simulink library "DodecaPreprocessingLib"  (R2020b)
settings: Solver=VariableStepAuto  StartTime=0.0  StopTime=10.0  RelTol=1e-3
undefined symbols (not defined in the file or in its folder): C_AccFiltCoeff, C_AngleScaleCoeff, C_DirectionTransmissionFactor, C_FiltStWhAngCoeff, C_FiltStWhAngSpdCoeff, C_Te_PPR, C_VehSpdCoeff, C_VspeedWfyaw, C_Wfyaw, C_WheelAxleDistance, N_AccMax, N_AccMin, N_ANGLES_N360_360, N_deg, N_max, N_min, N_pi, N_SIN_REL_N360_360, N_spd_conv
libraries: simulink x8, Valeo_Simulink_Library_EC x4
settings Model: Creator=ahashem  LastModifiedBy=ahashem

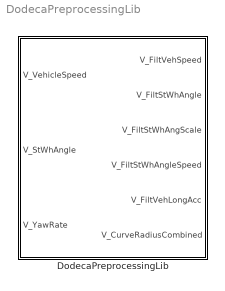
== system DodecaPreprocessingLib ==
  DodecaPreprocessingLib : Subsystem

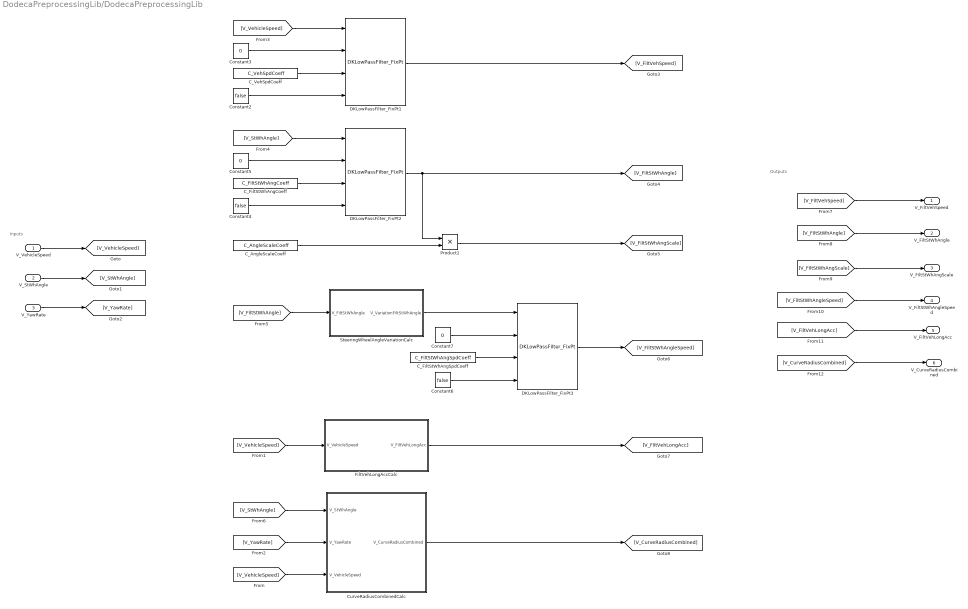
== system DodecaPreprocessingLib/DodecaPreprocessingLib ==
  note: Inputs
  note: Outputs
  V_VehicleSpeed : Inport  RequirementInfo={} %GIDa_60832143_23e3_4e37_9ef8_f4c8fbc195ea
  V_StWhAngle : Inport  RequirementInfo={} %GIDa_8126107c_488a_4046_91e4_66b596814474  Port=2
  V_YawRate : Inport  RequirementInfo={} %GIDa_21efb593_fe6a_4a8c_ad86_ea0a548e14f1  Port=3
  C_AngleScaleCoeff : Constant  RequirementInfo={} %GIDa_0cdad353_1e9f_40d8_8c36_6ad926c040fa  Value=C_AngleScaleCoeff  SampleTime=-1
  C_FiltStWhAngCoeff : Constant  RequirementInfo={} %GIDa_ea71535c_fca6_4d74_a353_bf553c7836cd  Value=C_FiltStWhAngCoeff  SampleTime=-1
  C_FiltStWhAngSpdCoeff : Constant  RequirementInfo={} %GIDa_088bdebb_9f79_46eb_9893_bd4dbe5423a2  Value=C_FiltStWhAngSpdCoeff  SampleTime=-1
  C_VehSpdCoeff : Constant  RequirementInfo={} %GIDa_c5f62ab8_0a9f_4fa0_82aa_9620af8d284b  Value=C_VehSpdCoeff  SampleTime=-1
  Constant2 : Constant  RequirementInfo={} %GIDa_f5b0f010_a49c_40bd_ade5_4da1f284b015  Value=false
  Constant3 : Constant  RequirementInfo={} %GIDa_bbc6fc55_9231_4124_a586_b78e3b3f8e3b  Value=0  OutDataTypeStr=Inherit: Inherit via back propagation
  Constant4 : Constant  RequirementInfo={} %GIDa_8db6b81b_f55b_4d76_a4c4_0f30a2bf3151  Value=false
  Constant5 : Constant  RequirementInfo={} %GIDa_1fff04a1_583c_4fc9_904f_aa895289aece  Value=0  OutDataTypeStr=Inherit: Inherit via back propagation
  Constant6 : Constant  RequirementInfo={} %GIDa_8cf859df_d5fb_4c8d_944a_ef0bb45c25e9  Value=false
  Constant7 : Constant  RequirementInfo={} %GIDa_d8cd6144_71a6_42bf_bf34_bb68e5da6881  Value=0  OutDataTypeStr=Inherit: Inherit via back propagation
  CurveRadiusCombinedCalc : Subsystem  RequirementInfo={} %GIDa_64336f43_2055_4d12_b781_db850783e38b
  DKLowPassFilter_FixPt1 : Valeo_Simulink_Library_EC/Signal_Operations/DKLowPassFilter_FixPt  Description=DKLowPassFilter_FixPt
  DKLowPassFilter_FixPt2 : Valeo_Simulink_Library_EC/Signal_Operations/DKLowPassFilter_FixPt  Description=DKLowPassFilter_FixPt
  DKLowPassFilter_FixPt3 : Valeo_Simulink_Library_EC/Signal_Operations/DKLowPassFilter_FixPt  Description=DKLowPassFilter_FixPt
  FiltVehLongAccCalc : Subsystem  RequirementInfo={} %GIDa_cd813895_0fe0_49b9_8029_c65e3c884f98  TreatAsAtomicUnit=on
  Product1 : Product  RequirementInfo={} %GIDa_f1608e0b_bb6d_46d5_89b0_19cc4592d5c7  OutDataTypeStr=Inherit: Inherit via back propagation  RndMeth=Round
  SteeringWheelAngleVariationCalc : Subsystem  RequirementInfo={} %GIDa_4c57f141_03ad_4307_827e_b71fe2f80d30
  V_FiltVehSpeed : Outport  RequirementInfo={} %GIDa_d767c948_d5f1_431d_a4d9_613e959d2370  VectorParamsAs1DForOutWhenUnconnected=off
  V_FiltStWhAngle : Outport  RequirementInfo={} %GIDa_20373fde_4aa9_40e5_8d80_7fd2414d965e  Port=2  VectorParamsAs1DForOutWhenUnconnected=off
  V_FiltStWhAngScale : Outport  RequirementInfo={} %GIDa_acd3b80a_9b27_4971_9a5d_d5919bd05f96  Port=3  VectorParamsAs1DForOutWhenUnconnected=off
  V_FiltStWhAngleSpeed : Outport  RequirementInfo={} %GIDa_08f10f9a_4278_41b2_90be_4b2c7de53d89  Port=4  VectorParamsAs1DForOutWhenUnconnected=off
  V_FiltVehLongAcc : Outport  RequirementInfo={} %GIDa_a987007b_cd5d_4cab_a6be_c6cc0e461b96  Port=5  VectorParamsAs1DForOutWhenUnconnected=off
  V_CurveRadiusCombined : Outport  RequirementInfo={} %GIDa_3bd352f3_c991_4ae8_b955_130684fa25fc  Port=6  VectorParamsAs1DForOutWhenUnconnected=off
  wires:
  V_VehicleSpeed/1 -> [V_VehicleSpeed]
  DKLowPassFilter_FixPt2/1 -> [V_FiltStWhAngle], Product1/1
  DKLowPassFilter_FixPt3/1 -> [V_FiltStWhAngleSpeed]
  V_YawRate/1 -> [V_YawRate]
  C_FiltStWhAngCoeff/1 -> DKLowPassFilter_FixPt2/3
  Constant7/1 -> DKLowPassFilter_FixPt3/2
  CurveRadiusCombinedCalc/1(V_CurveRadiusCombined) -> [V_CurveRadiusCombined]
  SteeringWheelAngleVariationCalc/1(V_VariationFiltStWhAngle) -> DKLowPassFilter_FixPt3/1
  Constant3/1 -> DKLowPassFilter_FixPt1/2
  [V_FiltStWhAngScale] -> V_FiltStWhAngScale/1
  [V_VehicleSpeed] -> FiltVehLongAccCalc/1(V_VehicleSpeed)
  [V_CurveRadiusCombined] -> V_CurveRadiusCombined/1
  [V_FiltVehLongAcc] -> V_FiltVehLongAcc/1
  [V_FiltStWhAngle] -> V_FiltStWhAngle/1
  [V_VehicleSpeed] -> CurveRadiusCombinedCalc/3(V_VehicleSpeed)
  Constant5/1 -> DKLowPassFilter_FixPt2/2
  [V_FiltVehSpeed] -> V_FiltVehSpeed/1
  [V_StWhAngle] -> CurveRadiusCombinedCalc/1(V_StWhAngle)
  FiltVehLongAccCalc/1(V_FiltVehLongAcc) -> [V_FiltVehLongAcc]
  [V_YawRate] -> CurveRadiusCombinedCalc/2(V_YawRate)
  Product1/1 -> [V_FiltStWhAngScale]
  V_StWhAngle/1 -> [V_StWhAngle]
  [V_FiltStWhAngle] -> SteeringWheelAngleVariationCalc/1(V_FiltStWhAngle)
  Constant4/1 -> DKLowPassFilter_FixPt2/4
  DKLowPassFilter_FixPt1/1 -> [V_FiltVehSpeed]
  Constant6/1 -> DKLowPassFilter_FixPt3/4
  [V_VehicleSpeed] -> DKLowPassFilter_FixPt1/1
  C_VehSpdCoeff/1 -> DKLowPassFilter_FixPt1/3
  [V_StWhAngle] -> DKLowPassFilter_FixPt2/1
  C_AngleScaleCoeff/1 -> Product1/2
  C_FiltStWhAngSpdCoeff/1 -> DKLowPassFilter_FixPt3/3
  Constant2/1 -> DKLowPassFilter_FixPt1/4
  [V_FiltStWhAngleSpeed] -> V_FiltStWhAngleSpeed/1

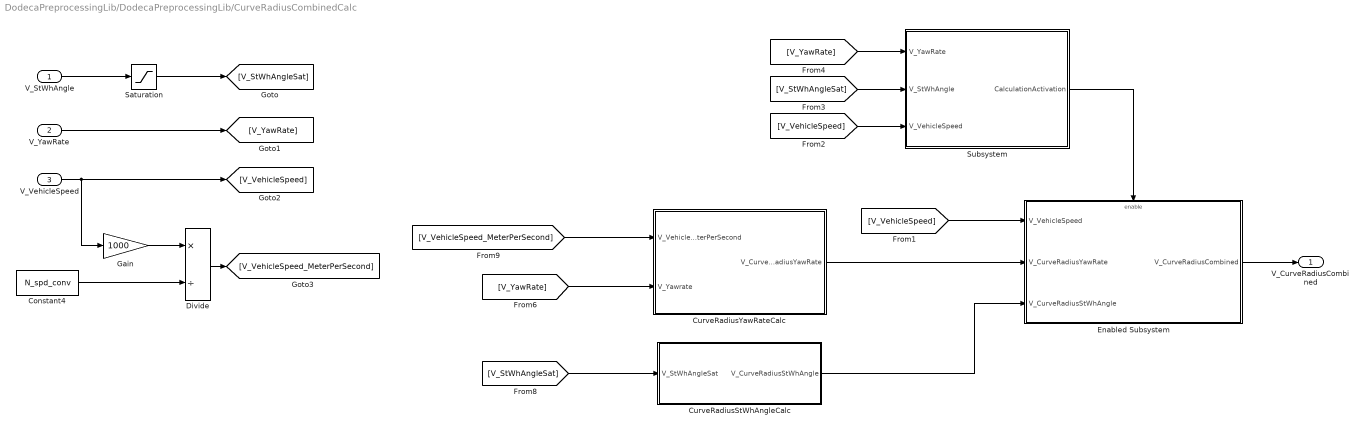
== system DodecaPreprocessingLib/DodecaPreprocessingLib/CurveRadiusCombinedCalc ==
  V_StWhAngle : Inport  RequirementInfo={} %GIDa_c6b31a6f_b3f8_4c38_b982_22111ad8ed9d
  V_YawRate : Inport  RequirementInfo={} %GIDa_7c4cc764_ca2d_41e9_9980_9d9fc3c311cd  Port=2
  V_VehicleSpeed : Inport  RequirementInfo={} %GIDa_23d1c370_e59f_4e6c_b1e1_69d048a5d2a4  Port=3
  Constant4 : Constant  RequirementInfo={} %GIDa_6504d488_faa2_46f4_83bf_1716aa9cad3c  Value=N_spd_conv
  CurveRadiusStWhAngleCalc : Subsystem  RequirementInfo={} %GIDa_d2b816be_039a_44fb_9baa_a094c55a53fb  TreatAsAtomicUnit=on
  CurveRadiusYawRateCalc : Subsystem  RequirementInfo={} %GIDa_2f2fda27_1e9c_44fd_a28d_c3986d892172  TreatAsAtomicUnit=on
  Divide : Product  RequirementInfo={} %GIDa_ae004ed8_02ea_45fd_a30c_5b5e6bbd11bf  Inputs=*/  RndMeth=Nearest
  Enabled Subsystem : Subsystem  RequirementInfo={} %GIDa_f954c3a3_b9a3_4728_bc26_2e3b533776b8  TreatAsAtomicUnit=on
  Gain : Gain  RequirementInfo={} %GIDa_717527a8_c330_4d57_a389_1cff86706634  Gain=1000  OutDataTypeStr=fixdt(1,32,0.01,0)
  Saturation : Saturate  RequirementInfo={} %GIDa_1b87c519_532e_4059_a469_dc5fcda7529d  UpperLimit=360  LowerLimit=-360  OutDataTypeStr=Inherit: Inherit via back propagation
  Subsystem : Subsystem  RequirementInfo={} %GIDa_2fc3370a_ff20_4ea0_b489_573f276c5142
  V_CurveRadiusCombined : Outport  RequirementInfo={} %GIDa_dbce3892_7d57_44c4_a2e6_0566f47b7bcf  VectorParamsAs1DForOutWhenUnconnected=off
  wires:
  Divide/1 -> [V_VehicleSpeed_MeterPerSecond]
  Constant4/1 -> Divide/2
  Gain/1 -> Divide/1
  V_VehicleSpeed/1 -> Gain/1, [V_VehicleSpeed]
  [V_StWhAngleSat] -> CurveRadiusStWhAngleCalc/1(V_StWhAngleSat)
  [V_YawRate] -> CurveRadiusYawRateCalc/2(V_Yawrate)
  [V_VehicleSpeed] -> Enabled Subsystem/1(V_VehicleSpeed)
  Subsystem/1(CalculationActivation) -> Enabled Subsystem/Enable
  [V_YawRate] -> Subsystem/1(V_YawRate)
  [V_StWhAngleSat] -> Subsystem/2(V_StWhAngle)
  [V_VehicleSpeed_MeterPerSecond] -> CurveRadiusYawRateCalc/1("V_VehicleSpeed_MeterPerSecond ")
  V_YawRate/1 -> [V_YawRate]
  Saturation/1 -> [V_StWhAngleSat]
  V_StWhAngle/1 -> Saturation/1
  CurveRadiusYawRateCalc/1(V_CurveRadiusYawRate) -> Enabled Subsystem/2(V_CurveRadiusYawRate)
  CurveRadiusStWhAngleCalc/1(V_CurveRadiusStWhAngle) -> Enabled Subsystem/3(V_CurveRadiusStWhAngle)
  Enabled Subsystem/1(V_CurveRadiusCombined) -> V_CurveRadiusCombined/1
  [V_VehicleSpeed] -> Subsystem/3(V_VehicleSpeed)

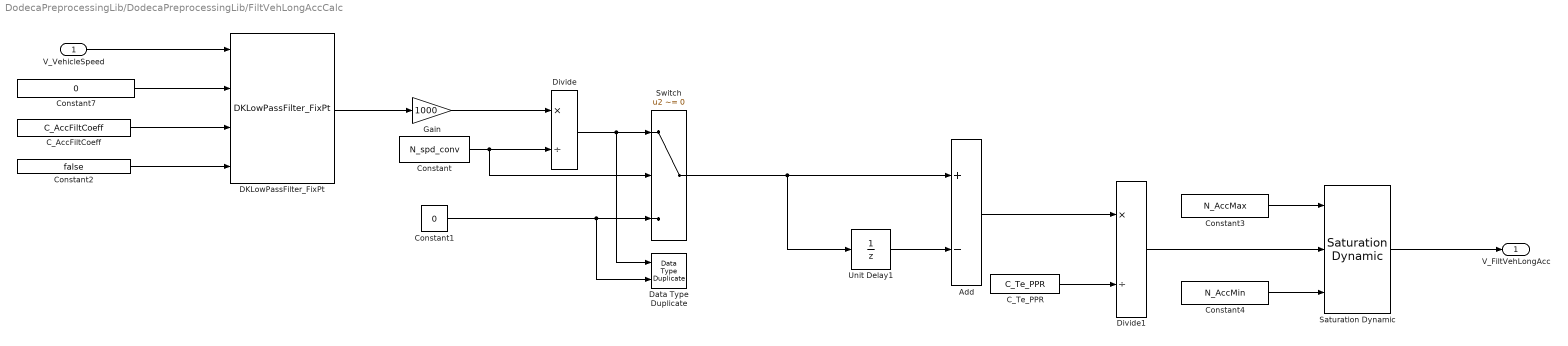
== system DodecaPreprocessingLib/DodecaPreprocessingLib/FiltVehLongAccCalc ==
  V_VehicleSpeed : Inport  RequirementInfo={} %GIDa_a9dff689_ed0f_4809_9958_382473ea2e53
  Add : Sum  RequirementInfo={} %GIDa_b5a1d6ae_d064_4547_8171_96b8d3b4d0ea  Inputs=+-  OutDataTypeStr=Inherit: Inherit via back propagation  RndMeth=Nearest
  C_AccFiltCoeff : Constant  RequirementInfo={} %GIDa_aac16ced_3053_42d0_a1c2_5613f13cadef  Value=C_AccFiltCoeff  SampleTime=-1
  C_Te_PPR : Constant  RequirementInfo={} %GIDa_ca0d0a07_9a87_4e79_85b6_5f4351a4e60f  Value=C_Te_PPR  SampleTime=-1
  Constant : Constant  RequirementInfo={} %GIDa_6440f10a_dfb1_4682_a064_f695864c14d3  Value=N_spd_conv
  Constant1 : Constant  RequirementInfo={} %GIDa_5e43bc7f_985f_4463_932e_96d3615ef032  Value=0  OutDataTypeStr=Inherit: Inherit via back propagation
  Constant2 : Constant  RequirementInfo={} %GIDa_ceee4a21_d10e_4212_9748_3affda2d37ce  Value=false
  Constant3 : Constant  RequirementInfo={} %GIDa_478474b1_827f_4edf_8a52_e111fe7d90da  Value=N_AccMax  VectorParams1D=off  SampleTime=-1
  Constant4 : Constant  RequirementInfo={} %GIDa_dd0b0e05_bb3a_4de4_bc6c_4a6892c59492  Value=N_AccMin  VectorParams1D=off  SampleTime=-1
  Constant7 : Constant  RequirementInfo={} %GIDa_4b056551_402d_41b4_8b01_4fbc664e95cb  Value=0  OutDataTypeStr=Inherit: Inherit via back propagation
  DKLowPassFilter_FixPt : Valeo_Simulink_Library_EC/Signal_Operations/DKLowPassFilter_FixPt  Description=DKLowPassFilter_FixPt
  Data Type Duplicate : DataTypeDuplicate  RequirementInfo={} %GIDa_d4dc3eef_3111_47ac_82d8_48f37c08ca8d
  Divide : Product  RequirementInfo={} %GIDa_2ebbd2e0_80ab_43ba_b182_82a6293abca0  Inputs=*/  RndMeth=Nearest  SaturateOnIntegerOverflow=on  OutDataTypeStr=Inherit: Same as first input
  Divide1 : Product  RequirementInfo={} %GIDa_2bef6155_8d7e_450c_988c_96a89a6309f6  Inputs=*/  OutDataTypeStr=Inherit: Inherit via back propagation  RndMeth=Nearest  SaturateOnIntegerOverflow=on
  Gain : Gain  RequirementInfo={} %GIDa_7eabfaa6_b6cc_4664_8175_45a7b4cb78a3  Gain=1000  OutDataTypeStr=fixdt(1,32,0.0005,0)  RndMeth=Nearest
  Saturation Dynamic : simulink/Discontinuities/Saturation Dynamic  OutMin=[]  OutMax=[]  OutDataTypeStr=fixdt(1,16,0.01,0)  OutputDataTypeScalingMode=Specify via dialog  OutDataType=fixdt(1,16,0.01,0)  OutScaling=[]  DoSatur=off
  Switch : Switch  RequirementInfo={} %GIDa_31131a59_f127_4858_9f67_3213aa90b36b  Criteria=u2 ~= 0
  Unit Delay1 : UnitDelay  RequirementInfo={} %GIDa_5fb9f8c5_fd76_4e8c_b532_a08efb54d5b6  SampleTime=-1  HasFrameUpgradeWarning=on
  V_FiltVehLongAcc : Outport  RequirementInfo={} %GIDa_1047f2a8_4318_4f33_b1e6_f10595ac80de  VectorParamsAs1DForOutWhenUnconnected=off
  wires:
  Constant1/1 -> Switch/3, Data Type Duplicate/2
  Divide/1 -> Switch/1, Data Type Duplicate/1
  Constant/1 -> Divide/2, Switch/2
  C_Te_PPR/1 -> Divide1/2
  Switch/1 -> Unit Delay1/1, Add/1
  Constant3/1 -> Saturation Dynamic/1
  Constant4/1 -> Saturation Dynamic/3
  Gain/1 -> Divide/1
  Add/1 -> Divide1/1
  Constant2/1 -> DKLowPassFilter_FixPt/4
  V_VehicleSpeed/1 -> DKLowPassFilter_FixPt/1
  C_AccFiltCoeff/1 -> DKLowPassFilter_FixPt/3
  Constant7/1 -> DKLowPassFilter_FixPt/2
  DKLowPassFilter_FixPt/1 -> Gain/1
  Unit Delay1/1 -> Add/2
  Divide1/1 -> Saturation Dynamic/2
  Saturation Dynamic/1 -> V_FiltVehLongAcc/1

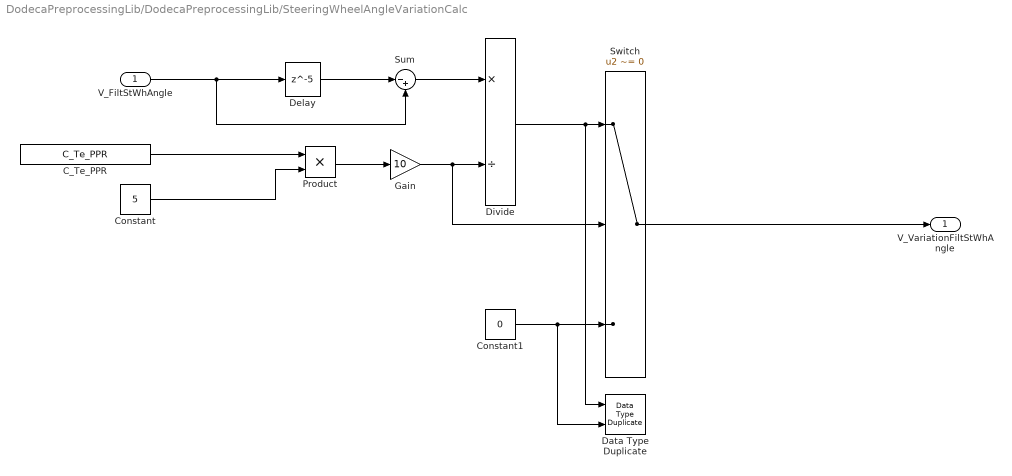
== system DodecaPreprocessingLib/DodecaPreprocessingLib/SteeringWheelAngleVariationCalc ==
  V_FiltStWhAngle : Inport  RequirementInfo={} %GIDa_2d6e10c8_a599_4818_8bca_4fdf95fdb51b
  C_Te_PPR : Constant  RequirementInfo={} %GIDa_d7d2a533_c78c_4824_bc3d_21d571249ced  Value=C_Te_PPR  SampleTime=-1
  Constant : Constant  RequirementInfo={} %GIDa_c4952c67_84f6_4782_887e_253009598a18  Value=5  OutDataTypeStr=uint8
  Constant1 : Constant  RequirementInfo={} %GIDa_c8535ef2_48fc_41db_9114_3d1e05bc0590  Value=0  OutDataTypeStr=Inherit: Inherit via back propagation
  Data Type Duplicate : DataTypeDuplicate  RequirementInfo={} %GIDa_92bb835e_761a_4655_8305_5c552c08e307
  Delay : Delay  RequirementInfo={} %GIDa_72bb8d93_5d0e_4efa_b41a_7b2f3ca524a6  DelayLength=5
  Divide : Product  RequirementInfo={} %GIDa_e876373c_7d20_4d9f_848c_1236b8df3224  Inputs=*/  OutDataTypeStr=Inherit: Inherit via back propagation  RndMeth=Nearest  SaturateOnIntegerOverflow=on
  Gain : Gain  RequirementInfo={} %GIDa_7bda443d_549c_42d1_a512_94fec012033d  Gain=10  OutDataTypeStr=Inherit: Same as input
  Product : Product  RequirementInfo={} %GIDa_d173abd4_ab08_494f_97f9_3c8702ce310b  OutDataTypeStr=Inherit: Same as first input
  Sum : Sum  RequirementInfo={} %GIDa_9d1cd385_e87c_41c8_a3c2_c3015445a319  Inputs=|-+  InputSameDT=on  SaturateOnIntegerOverflow=on  OutDataTypeStr=Inherit: Same as first input
  Switch : Switch  RequirementInfo={} %GIDa_fbe2b111_2dff_405a_b4e7_13e74d307d11  Criteria=u2 ~= 0
  V_VariationFiltStWhAngle : Outport  RequirementInfo={} %GIDa_7cff779a_541a_4368_a5cc_b4cb3fe5e430  VectorParamsAs1DForOutWhenUnconnected=off
  wires:
  Gain/1 -> Divide/2, Switch/2
  Product/1 -> Gain/1
  Switch/1 -> V_VariationFiltStWhAngle/1
  Divide/1 -> Switch/1, Data Type Duplicate/1
  Constant1/1 -> Switch/3, Data Type Duplicate/2
  C_Te_PPR/1 -> Product/1
  Constant/1 -> Product/2
  V_FiltStWhAngle/1 -> Sum/2, Delay/1
  Sum/1 -> Divide/1
  Delay/1 -> Sum/1

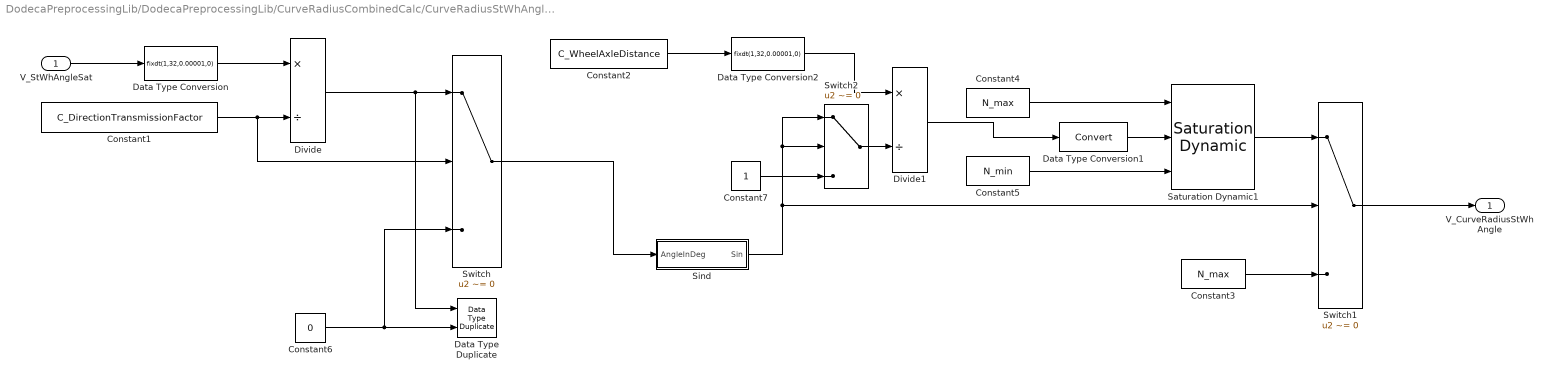
== system DodecaPreprocessingLib/DodecaPreprocessingLib/CurveRadiusCombinedCalc/CurveRadiusStWhAngleCalc ==
  V_StWhAngleSat : Inport  RequirementInfo={} %GIDa_abb681a8_9c5f_45e7_85c6_1a1dee86fac2
  Constant1 : Constant  RequirementInfo={} %GIDa_98570868_5dac_488f_8353_c0564531cf00  Value=C_DirectionTransmissionFactor
  Constant2 : Constant  RequirementInfo={} %GIDa_62b48d84_6a64_4fdc_8bb8_1a0424173a6d  Value=C_WheelAxleDistance
  Constant3 : Constant  Value=N_max
  Constant4 : Constant  RequirementInfo={} %GIDa_fa7813f2_9f7f_4d54_bbcf_f72d7c254580  Value=N_max
  Constant5 : Constant  RequirementInfo={} %GIDa_dd5c7f71_2632_4dc2_942f_60a3de9821df  Value=N_min
  Constant6 : Constant  RequirementInfo={} %GIDa_a1627ed7_883d_4f6e_b8c6_462b0de5ac4d  Value=0  OutDataTypeStr=Inherit: Inherit via back propagation
  Constant7 : Constant  OutDataTypeStr=Inherit: Inherit via back propagation
  Data Type Duplicate : DataTypeDuplicate  RequirementInfo={} %GIDa_9fb6f9e2_a828_4c5c_bf89_f0860357c30f
  Data Type Conversion : DataTypeConversion  RequirementInfo={} %GIDa_2b46cdeb_753e_4edf_9749_a9910cb6b44c  OutDataTypeStr=fixdt(1,32,0.00001,0)
  Data Type Conversion1 : DataTypeConversion  RequirementInfo={} %GIDa_3c386ddb_68dc_423b_897b_b241bf86d79b  RndMeth=Nearest
  Data Type Conversion2 : DataTypeConversion  RequirementInfo={} %GIDa_3ec3c6aa_b003_4747_bc1a_e15dfe0f1686  OutDataTypeStr=fixdt(1,32,0.00001,0)
  Divide : Product  RequirementInfo={} %GIDa_6c6f0a1c_13d3_4619_9e0e_e7ddaa12e435  Inputs=*/  RndMeth=Nearest  SaturateOnIntegerOverflow=on  OutDataTypeStr=Inherit: Same as first input
  Divide1 : Product  RequirementInfo={} %GIDa_1850e6e0_24fb_4802_a9cd_363db8f8d411  Inputs=*/  RndMeth=Nearest  SaturateOnIntegerOverflow=on  OutDataTypeStr=Inherit: Same as first input
  Saturation Dynamic1 : simulink/Discontinuities/Saturation Dynamic  OutMin=[]  OutMax=[]  OutDataTypeStr=int16  OutputDataTypeScalingMode=int16  OutDataType=fixdt(1, 16)  OutScaling=2^-10  DoSatur=off
  Sind : Subsystem  RequirementInfo={} %GIDa_c2fe74d6_4e4e_4053_a67d_4d963e843008
  Switch : Switch  RequirementInfo={} %GIDa_946765d4_88f0_459a_88a2_95c5b5a25c8b  Criteria=u2 ~= 0
  Switch1 : Switch  RequirementInfo={} %GIDa_9d5e6c70_41f5_4b04_9d9f_b48aab403a01  Criteria=u2 ~= 0
  Switch2 : Switch  Criteria=u2 ~= 0
  V_CurveRadiusStWhAngle : Outport  RequirementInfo={} %GIDa_d4150f61_a977_42d0_8013_f59b9b8bd2a2  VectorParamsAs1DForOutWhenUnconnected=off
  wires:
  Data Type Conversion1/1 -> Saturation Dynamic1/2
  Switch1/1 -> V_CurveRadiusStWhAngle/1
  Saturation Dynamic1/1 -> Switch1/1
  Divide1/1 -> Data Type Conversion1/1
  Data Type Conversion2/1 -> Divide1/1
  Constant1/1 -> Divide/2, Switch/2
  Data Type Conversion/1 -> Divide/1
  Divide/1 -> Data Type Duplicate/1, Switch/1
  Constant6/1 -> Switch/3, Data Type Duplicate/2
  Constant5/1 -> Saturation Dynamic1/3
  Constant4/1 -> Saturation Dynamic1/1
  Switch/1 -> Sind/1(AngleInDeg)
  V_StWhAngleSat/1 -> Data Type Conversion/1
  Constant2/1 -> Data Type Conversion2/1
  Sind/1(Sin) -> Switch2/1, Switch2/2, Switch1/2
  Constant3/1 -> Switch1/3
  Switch2/1 -> Divide1/2
  Constant7/1 -> Switch2/3

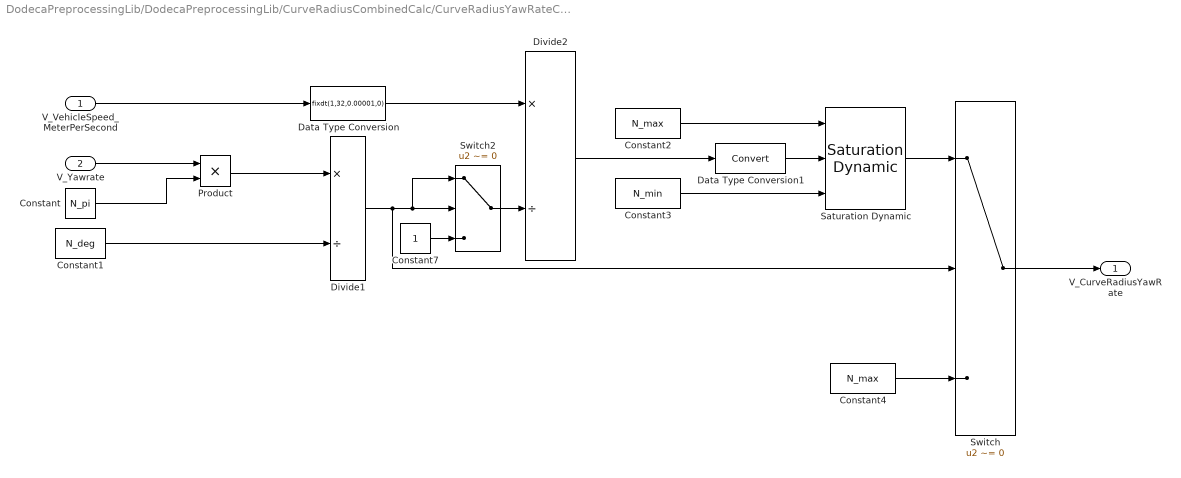
== system DodecaPreprocessingLib/DodecaPreprocessingLib/CurveRadiusCombinedCalc/CurveRadiusYawRateCalc ==
  "V_VehicleSpeed_MeterPerSecond " : Inport  RequirementInfo={} %GIDa_b8150515_5fed_43e7_a020_4c3dd0662e2c
  V_Yawrate : Inport  RequirementInfo={} %GIDa_a8c62ac7_f65c_41a8_8300_229a5a8f87bd  Port=2
  Constant : Constant  RequirementInfo={} %GIDa_5cc06acd_85f2_41c2_868f_dd9dcb282a6d  Value=N_pi
  Constant1 : Constant  RequirementInfo={} %GIDa_0439bdf0_1d9d_4128_851a_8e4062f2ea6e  Value=N_deg
  Constant2 : Constant  RequirementInfo={} %GIDa_9d31224f_c4e5_4964_84c0_bdb99a5399a4  Value=N_max
  Constant3 : Constant  RequirementInfo={} %GIDa_b839a59b_1189_4377_b595_5dfb5ba75ca6  Value=N_min
  Constant4 : Constant  Value=N_max
  Constant7 : Constant  OutDataTypeStr=Inherit: Inherit via back propagation
  Data Type Conversion : DataTypeConversion  RequirementInfo={} %GIDa_bb5325b8_eece_4956_a4e1_c3c780cceb19  OutDataTypeStr=fixdt(1,32,0.00001,0)  RndMeth=Nearest
  Data Type Conversion1 : DataTypeConversion  RequirementInfo={} %GIDa_b72d1d93_d1e7_44eb_9859_a7d629f5b22f  RndMeth=Nearest
  Divide1 : Product  RequirementInfo={} %GIDa_c4f2fba1_a6dc_479b_859e_320a67e827c4  Inputs=*/  RndMeth=Nearest  OutDataTypeStr=Inherit: Same as first input
  Divide2 : Product  RequirementInfo={} %GIDa_3edd98d5_7516_4631_93a5_dc5abed02e4a  Inputs=*/  RndMeth=Nearest  SaturateOnIntegerOverflow=on  OutDataTypeStr=Inherit: Same as first input
  Product : Product  RequirementInfo={} %GIDa_deeedb41_50b5_400e_a3b1_edb035b115c2  OutDataTypeStr=fixdt(1,32,0.00001,0)  RndMeth=Nearest
  Saturation Dynamic : simulink/Discontinuities/Saturation Dynamic  OutMin=[]  OutMax=[]  OutDataTypeStr=int16  OutputDataTypeScalingMode=int16  OutDataType=fixdt(1, 16)  OutScaling=2^-10  DoSatur=off
  Switch : Switch  RequirementInfo={} %GIDa_9386fa3b_9e9d_48a1_80ed_e0e569d2533b  Criteria=u2 ~= 0
  Switch2 : Switch  Criteria=u2 ~= 0
  V_CurveRadiusYawRate : Outport  RequirementInfo={} %GIDa_8a4eb58c_61b4_43a7_81c7_927a1839a6fd  VectorParamsAs1DForOutWhenUnconnected=off
  wires:
  Data Type Conversion1/1 -> Saturation Dynamic/2
  Saturation Dynamic/1 -> Switch/1
  Switch/1 -> V_CurveRadiusYawRate/1
  V_Yawrate/1 -> Product/1
  Divide2/1 -> Data Type Conversion1/1
  Data Type Conversion/1 -> Divide2/1
  "V_VehicleSpeed_MeterPerSecond "/1 -> Data Type Conversion/1
  Constant2/1 -> Saturation Dynamic/1
  Constant3/1 -> Saturation Dynamic/3
  Product/1 -> Divide1/1
  Constant/1 -> Product/2
  Constant1/1 -> Divide1/2
  Constant4/1 -> Switch/3
  Divide1/1 -> Switch2/1, Switch2/2, Switch/2
  Constant7/1 -> Switch2/3
  Switch2/1 -> Divide2/2

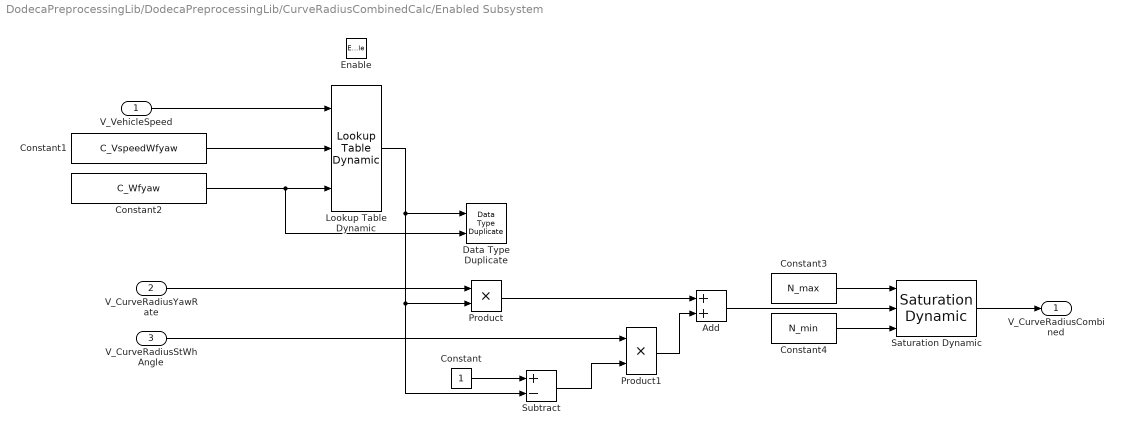
== system DodecaPreprocessingLib/DodecaPreprocessingLib/CurveRadiusCombinedCalc/Enabled Subsystem ==
  V_VehicleSpeed : Inport  RequirementInfo={} %GIDa_d0a89e53_c69c_48c6_be63_657fcb00fd51
  V_CurveRadiusYawRate : Inport  RequirementInfo={} %GIDa_7f9f37da_4753_4ff2_b91a_6ca43b5994df  Port=2
  V_CurveRadiusStWhAngle : Inport  RequirementInfo={} %GIDa_e774cc64_851a_4925_9b06_1482a75aec84  Port=3
  Enable : EnablePort  RequirementInfo={} %GIDa_89b4ce9b_cb09_4e0b_90d9_aeaddfbaca67
  Add : Sum  RequirementInfo={} %GIDa_55cc3eda_696f_41cb_8001_616f030fd0d5  AccumDataTypeStr=int16
  Constant : Constant  RequirementInfo={} %GIDa_e4604bdc_ac83_48c8_b31d_fce12cb68eff  OutDataTypeStr=Inherit: Inherit via back propagation
  Constant1 : Constant  RequirementInfo={} %GIDa_22c38c13_3950_405b_9b2e_515dac8b5bfb  Value=C_VspeedWfyaw  OutDataTypeStr=Inherit: Inherit via back propagation
  Constant2 : Constant  RequirementInfo={} %GIDa_e19677ab_1ab0_4527_924f_5d5d4d55dec3  Value=C_Wfyaw
  Constant3 : Constant  RequirementInfo={} %GIDa_26c23a02_aa05_432d_ae1f_c0fda192a889  Value=N_max
  Constant4 : Constant  RequirementInfo={} %GIDa_a9f86592_ef25_41bc_ba65_2d1f866949e0  Value=N_min
  Data Type Duplicate : DataTypeDuplicate  RequirementInfo={} %GIDa_1a562d00_aff2_46e1_9c5b_b125180d00d3
  Lookup Table Dynamic : simulink/Lookup Tables/Lookup Table Dynamic  LookUpMeth=Interpolation-Use End Values  OutDataType=fixdt('uint8')  OutScaling=[]  OutDataTypeStr=Inherit: Inherit via back propagation  RndMeth=Nearest  DoSatur=off
  Product : Product  RequirementInfo={} %GIDa_cebdd8bd_3ab2_4290_9634_fc4191a4e391  OutDataTypeStr=int16
  Product1 : Product  RequirementInfo={} %GIDa_0cad0d15_a045_4abe_bf99_1dfb14ec51f1  OutDataTypeStr=int16
  Saturation Dynamic : simulink/Discontinuities/Saturation Dynamic  OutMin=[]  OutMax=[]  OutDataTypeStr=Inherit: Same as second input  OutDataType=fixdt(1, 16)  OutScaling=2^-10  DoSatur=off
  Subtract : Sum  RequirementInfo={} %GIDa_6a0dda27_47f4_41f6_bf61_356e686d6cc7  Inputs=+-
  V_CurveRadiusCombined : Outport  RequirementInfo={} %GIDa_dfda7476_d96b_48f1_8302_2de1f61a3e3d  VectorParamsAs1DForOutWhenUnconnected=off
  wires:
  Lookup Table Dynamic/1 -> Data Type Duplicate/1, Product/2, Subtract/2
  Constant1/1 -> Lookup Table Dynamic/2
  V_VehicleSpeed/1 -> Lookup Table Dynamic/1
  Constant2/1 -> Data Type Duplicate/2, Lookup Table Dynamic/3
  Constant/1 -> Subtract/1
  Product/1 -> Add/1
  Product1/1 -> Add/2
  Saturation Dynamic/1 -> V_CurveRadiusCombined/1
  Constant3/1 -> Saturation Dynamic/1
  Constant4/1 -> Saturation Dynamic/3
  Add/1 -> Saturation Dynamic/2
  V_CurveRadiusYawRate/1 -> Product/1
  Subtract/1 -> Product1/2
  V_CurveRadiusStWhAngle/1 -> Product1/1

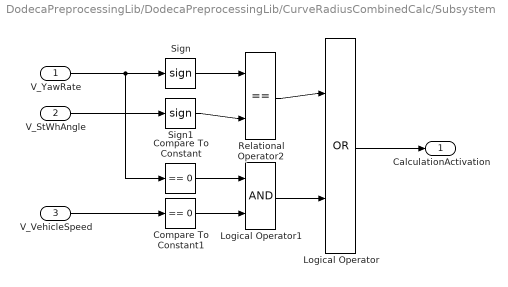
== system DodecaPreprocessingLib/DodecaPreprocessingLib/CurveRadiusCombinedCalc/Subsystem ==
  V_YawRate : Inport  RequirementInfo={} %GIDa_90b60cdc_1b49_49d0_bb9c_c81c08584575
  V_StWhAngle : Inport  RequirementInfo={} %GIDa_5d093c7e_f779_451b_95cd_bc6afae4231a  Port=2
  V_VehicleSpeed : Inport  Port=3
  Compare To Constant : simulink/Logic and Bit Operations/Compare To Constant  relop===  const=0  OutDataTypeStr=boolean
  Compare To Constant1 : simulink/Logic and Bit Operations/Compare To Constant  relop===  const=0  OutDataTypeStr=boolean
  Logical Operator : Logic  RequirementInfo={} %GIDa_5e501473_f971_4112_8641_f9d75db1b138  Operator=OR  AllPortsSameDT=off  OutDataTypeStr=boolean
  Logical Operator1 : Logic  AllPortsSameDT=off  OutDataTypeStr=boolean
  Relational Operator2 : RelationalOperator  RequirementInfo={} %GIDa_7c94afc0_7b84_479d_9881_a6c18374c079  Operator===  OutDataTypeStr=boolean  RndMeth=Simplest
  Sign : Signum  RequirementInfo={} %GIDa_2c291c99_6318_467a_a7ef_0bd69f6c9d21
  Sign1 : Signum  RequirementInfo={} %GIDa_8d3bf92a_536c_42bb_a261_542d172f4bea
  CalculationActivation : Outport  RequirementInfo={} %GIDa_74669a86_fbb9_4ad3_bce0_9a40e3ffe63a  VectorParamsAs1DForOutWhenUnconnected=off
  wires:
  V_StWhAngle/1 -> Sign1/1
  Logical Operator/1 -> CalculationActivation/1
  Sign1/1 -> Relational Operator2/2
  V_YawRate/1 -> Compare To Constant/1, Sign/1
  Sign/1 -> Relational Operator2/1
  Relational Operator2/1 -> Logical Operator/1
  Logical Operator1/1 -> Logical Operator/2
  Compare To Constant/1 -> Logical Operator1/1
  V_VehicleSpeed/1 -> Compare To Constant1/1
  Compare To Constant1/1 -> Logical Operator1/2

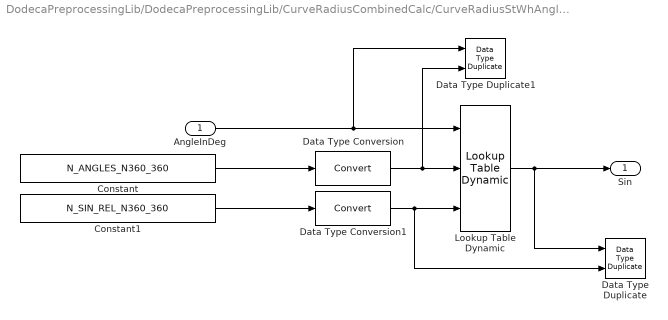
== system DodecaPreprocessingLib/DodecaPreprocessingLib/CurveRadiusCombinedCalc/CurveRadiusStWhAngleCalc/Sind ==
  AngleInDeg : Inport  RequirementInfo={} %GIDa_5d43a642_21c1_4c4d_b51c_58c61953a24a
      settings: AttributesFormatString=%<OutDataTypeStr>
  Constant : Constant  RequirementInfo={} %GIDa_016ba24c_9318_4898_af25_ce89615eee45  Value=N_ANGLES_N360_360
  Constant1 : Constant  RequirementInfo={} %GIDa_37d4dbb4_240a_4a1c_b050_6d29506b8652  Value=N_SIN_REL_N360_360
  Data Type Duplicate : DataTypeDuplicate  RequirementInfo={} %GIDa_f23523d7_d670_4cf6_be28_bea5a261487e
  Data Type Duplicate1 : DataTypeDuplicate  RequirementInfo={} %GIDa_7c850d2e_fe86_492a_92ea_be77173110d9
  Data Type Conversion : DataTypeConversion  RequirementInfo={} %GIDa_134b382e_36af_40af_8776_f39b3d743c67
  Data Type Conversion1 : DataTypeConversion  RequirementInfo={} %GIDa_ce57439a_3f10_4d2c_bc6c_618fa6518e37
  Lookup Table Dynamic : simulink/Lookup Tables/Lookup Table Dynamic  LookUpMeth=Interpolation-Use End Values  OutDataType=fixdt(1,32,0.0001,0)  OutScaling=[]  OutDataTypeStr=Inherit: Inherit via back propagation  RndMeth=Nearest  DoSatur=off
  Sin : Outport  RequirementInfo={} %GIDa_1d9909cb_d88c_441a_a4ef_d908fd2874db  VectorParamsAs1DForOutWhenUnconnected=off
      settings: AttributesFormatString=%<OutDataTypeStr>
  wires:
  Lookup Table Dynamic/1 -> Data Type Duplicate/1, Sin/1
  Constant/1 -> Data Type Conversion/1
  Constant1/1 -> Data Type Conversion1/1
  AngleInDeg/1 -> Lookup Table Dynamic/1, Data Type Duplicate1/1
  Data Type Conversion/1 -> Data Type Duplicate1/2, Lookup Table Dynamic/2
  Data Type Conversion1/1 -> Data Type Duplicate/2, Lookup Table Dynamic/3
